simulink model "BalancingRobotSS"  (R2022b)
settings: Solver=ode15s  StartTime=0.0  StopTime=60  FixedStep=0.01  RelTol=1e-3
values from neighbouring files (symbols this model uses):
  drv =     [parameters.mat]
  gbox =     [parameters.mat]
  sens =     [parameters.mat]
  Ts = 1e-2    (= 0.01)    [DataLAB4.m]    (also in parameters.mat)
  wheel =     [parameters.mat]
undefined symbols (not defined in the file or in its folder): controller, DiscIntNeverNeededParam, filt, yaw
settings Model: Creator=Alessandro  LastModifiedBy=perondavid
settings SolverCC: AlgebraicLoopSolver=TrustRegion
settings ModelReferenceCC: EnableRefExpFcnMdlSchedulingChecks=on
settings RTWCC: DLArmComputeVersion=19.05

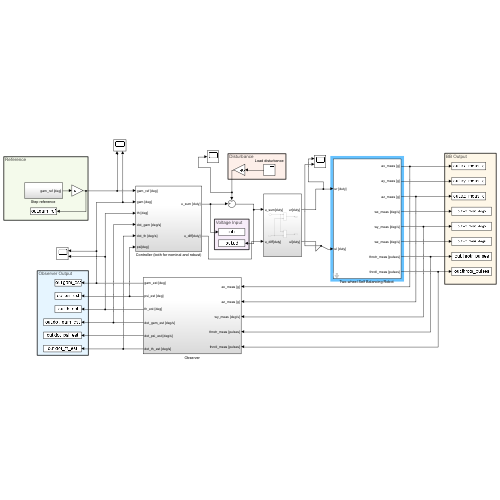
[thumbnail: Simulink's stored preview of the top-level diagram]
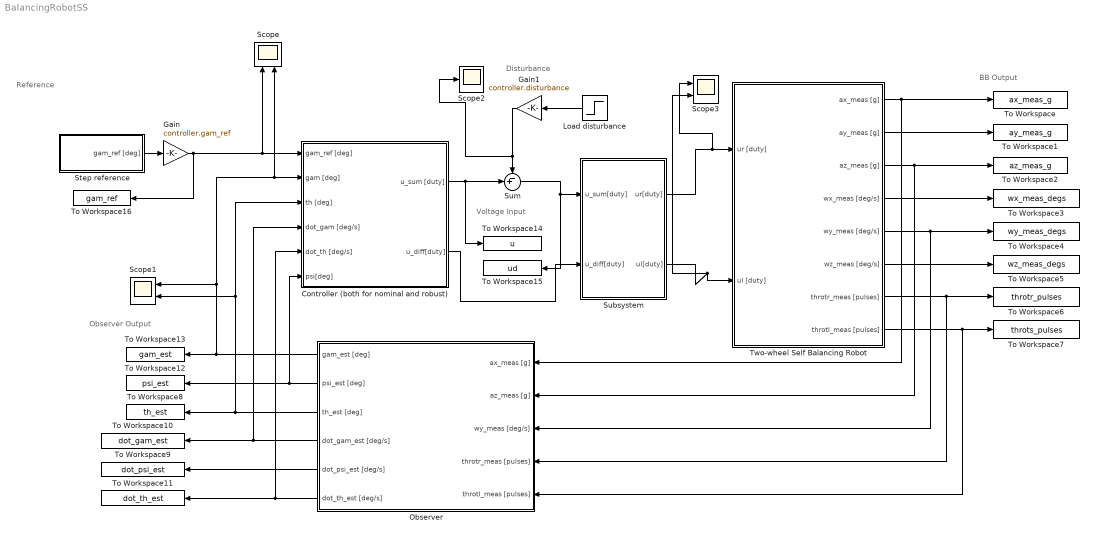
== system BalancingRobotSS ==
  note: Disturbance
  note: Reference
  note: Voltage Input
  note: Observer Output
  note: BB Output
  Controller (both for nominal and robust) : Subsystem
  Gain : Gain  Gain=controller.gam_ref
  Gain1 : Gain  Gain=controller.disturbance
  Load disturbance : Step  Time=10  After=5.0/drv.duty2V  SampleTime=Ts  VectorParams1D=off
  Observer : Subsystem
  Scope : Scope  NumInputPorts=2
  Scope1 : Scope  NumInputPorts=2
  Scope2 : Scope
  Scope3 : Scope  NumInputPorts=2
  "Step reference " : Subsystem
  Subsystem : Subsystem
  Sum : Sum  Inputs=-+|
  To Workspace : ToWorkspace  VariableName=ax_meas_g  SaveFormat=Structure With Time  SampleTime=-1
  To Workspace1 : ToWorkspace  VariableName=ay_meas_g  SaveFormat=Structure With Time  SampleTime=-1
  To Workspace10 : ToWorkspace  VariableName=dot_gam_est  SaveFormat=Structure With Time  SampleTime=-1
  To Workspace11 : ToWorkspace  VariableName=dot_th_est  SaveFormat=Structure With Time  SampleTime=-1
  To Workspace12 : ToWorkspace  VariableName=psi_est  SaveFormat=Structure With Time  SampleTime=-1
  To Workspace13 : ToWorkspace  VariableName=gam_est  SaveFormat=Structure With Time  SampleTime=-1
  To Workspace14 : ToWorkspace  VariableName=u  SaveFormat=Structure With Time  SampleTime=-1
  To Workspace15 : ToWorkspace  VariableName=ud  SaveFormat=Structure With Time  SampleTime=-1
  To Workspace16 : ToWorkspace  VariableName=gam_ref  SaveFormat=Structure With Time  SampleTime=-1
  To Workspace2 : ToWorkspace  VariableName=az_meas_g  SaveFormat=Structure With Time  SampleTime=-1
  To Workspace3 : ToWorkspace  VariableName=wx_meas_degs  SaveFormat=Structure With Time  SampleTime=-1
  To Workspace4 : ToWorkspace  VariableName=wy_meas_degs  SaveFormat=Structure With Time  SampleTime=-1
  To Workspace5 : ToWorkspace  VariableName=wz_meas_degs  SaveFormat=Structure With Time  SampleTime=-1
  To Workspace6 : ToWorkspace  VariableName=throtr_pulses  SaveFormat=Structure With Time  SampleTime=-1
  To Workspace7 : ToWorkspace  VariableName=throts_pulses  SaveFormat=Structure With Time  SampleTime=-1
  To Workspace8 : ToWorkspace  VariableName=th_est  SaveFormat=Structure With Time  SampleTime=-1
  To Workspace9 : ToWorkspace  VariableName=dot_psi_est  SaveFormat=Structure With Time  SampleTime=-1
  "Two-wheel Self Balancing Robot " : Subsystem  mask(Balancing robot (longitudinal + lateral dynamics)){initState=[0, 0, 0, 0, 0, 0], Ts=Ts}
      mask prompts: initState "Initial state [gam(0), psi(0), th(0), dot_gam(0), dot_psi(0), dot_th(0)]'"; Ts "Sample time:"
      mask help:
      | Balancing robot dynamic model.
      | Includes both the longitudinal and lateral (yaw) dynamics.
      mask init:
      | %% General parameters and conversion gains
      | 
      | %   gravity acc [m/s^2]
      | g = 9.81;
      | 
      | %   conversion gains
      | rpm2rads = 2*pi/60;         %   [rpm]   -> [rad/s]
      | rads2rpm = 60/2/pi;         %   [rad/s] -> [rpm]
      | rpm2degs = 360/60;          %   [rpm]   -> [deg/s]
      | degs2rpm = 60/360;          %   [deg/s] -> [rpm]
      | deg2rad = pi/180;           %   [deg]   -> [rad]
      | rad2deg = 180/pi;           %   [rad]   -> [deg]
      | g2ms2 = g;                  %   [acc_g] -> [m/s^2]
      | ms22g = 1/g;                %   [m/s^2] -> [acc_g]
      | ozin2Nm = 0.706e-2;         %   [oz*inch] -> [N*m]
      | 
      | 
      | %%  Battery data
      | 
      | %   electrical data
      | batt.UN = 11.1;     %   nominal voltage
      | 
      | 
      | %%  H-bridge PWM voltage driver
      | 
      | drv.Vbus = batt.UN;                     %   H-bridge DC bus voltage  
      | drv.pwm.bits = 8;                       %   PWM resolution [bits]
      | drv.pwm.levels = 2^drv.pwm.bits;        %   PWM levels
      | drv.pwm.Fs = 490;                       %   PWM frequency
      | drv.dutymax = drv.pwm.levels-1;         %   max duty cycle code
      | drv.duty2V = drv.Vbus/drv.dutymax;      %   duty cycle code (0-255) to voltage
      | drv.V2duty = drv.dutymax/drv.Vbus;      %   voltage to duty cycle code (0-255)
      | 
      | 
      | %%  Gearbox data 
      | 
      | gbox.N = 30;            %   reduction ratio
      | 
      | 
      | %%  Sensors data - Hall-effect encoder
      | 
      | %   Hall-effect encoder
      | sens.enc.ppr = 16*4;    %   pulses per rotation at motor side (w/ quadrature decoding)
      | sens.enc.pulse2deg = 360/sens.enc.ppr;
      | sens.enc.pulse2rad = 2*pi/sens.enc.ppr;
      | sens.enc.deg2pulse = sens.enc.ppr/360;
      | sens.enc.rad2pulse = sens.enc.ppr/2/pi;
      | 
      | 
      | %%  Sensors data - MPU6050 (accelerometer + gyro)
      | 
      | %   center of mass (CoM) position
      | sens.mpu.xb = 0;
      | sens.mpu.yb = 0;
      | sens.mpu.zb = 13.5e-3;
      | 
      | %       MPU6050 embedded accelerometer specs
      | sens.mpu.acc.bits = 16;
      | sens.mpu.acc.fs_g = 16;                                                         %   full-scale in "g" units
      | sens.mpu.acc.fs = sens.mpu.acc.fs_g * g2ms2;                                    %   full-scale in [m/s^2] 
      | sens.mpu.acc.g2LSB = floor(2^(sens.mpu.acc.bits-1)/sens.mpu.acc.fs_g);          %   sensitivity [LSB/g]
      | sens.mpu.acc.ms22LSB = sens.mpu.acc.g2LSB * ms22g;                              %   sensitvity [LSB/(m/s^2)]
      | sens.mpu.acc.LSB2g = sens.mpu.acc.fs_g/2^(sens.mpu.acc.bits-1);                 %   output quantization step [g/LSB]
      | sens.mpu.acc.LSB2ms2 = sens.mpu.acc.LSB2g * g2ms2;                              %   output quantization step [ms2/LSB]
      | sens.mpu.acc.bw = 94;                                                           %   output low-pass filter bandwidth
      | sens.mpu.acc.noisestd = 400e-6*sqrt(100);                                       %   output noise std [g-rms]
      | sens.mpu.acc.noisevar = sens.mpu.acc.noisestd^2;                                %   output noise var [g^2]
      | 
      | %       MPU6050 embdedded gyroscope specs
      | sens.mpu.gyro.bits = 16;
      | sens.mpu.gyro.fs_degs = 250;                                                    %   full scale in [deg/s (dps)]
      | sens.mpu.gyro.fs = sens.mpu.gyro.fs_degs * deg2rad;                             %   full scale in [rad/s]
      | sens.mpu.gyro.degs2LSB = floor(2^(sens.mpu.gyro.bits-1)/sens.mpu.gyro.fs_degs);	%   sensitivity [LSB/degs]
      | sens.mpu.gyro.rads2LSB = sens.mpu.gyro.degs2LSB * rad2deg;                      %   sensitivity [LSB/rads] 
      | sens.mpu.gyro.LSB2degs = sens.mpu.gyro.fs_degs/2^(sens.mpu.gyro.bits-1);        %   output quantization step [degs/LSB]
      | sens.mpu.gyro.LSB2rads = sens.mpu.gyro.LSB2degs * deg2rad;                      %   output quantization step [rads/LSB]
      | sens.mpu.gyro.bw = 98;                                                          %   output low-pass filter bandwidth
      | sens.mpu.gyro.noisestd = 5e-3*sqrt(100);                                        %   output noise std [degs-rms]
      | sens.mpu.gyro.noisevar = sens.mpu.acc.noisestd ^2;                              %   output noise var [degs^2]
      mask Help:
      | Riccardo Antonello (antonello@dei.unipd.it)
      | 
      | May 19, 2020
      | 
      | Dept. of Information Engineering, University of Padova
  wires:
  Controller (both for nominal and robust)/1(u_sum [duty]) -> To Workspace14/1, Sum/2
  Observer/1(gam_est [deg]) -> Scope1/1, Scope/2, Controller (both for nominal and robust)/2(gam [deg]), To Workspace13/1
  Sum/1 -> To Workspace15/1, Subsystem/1(u_sum[duty])
  "Two-wheel Self Balancing Robot "/2(ay_meas [g]) -> To Workspace1/1
  "Two-wheel Self Balancing Robot "/4(wx_meas [deg/s]) -> To Workspace3/1
  "Two-wheel Self Balancing Robot "/6(wz_meas [deg/s]) -> To Workspace5/1
  Observer/3(th_est [deg]) -> To Workspace8/1, Scope1/2, Controller (both for nominal and robust)/3(th [deg])
  Observer/6(dot_th_est [deg/s]) -> Controller (both for nominal and robust)/5(dot_th [deg/s]), To Workspace11/1
  Observer/5(dot_psi_est [deg/s]) -> To Workspace9/1
  Load disturbance/1 -> Gain1/1
  "Two-wheel Self Balancing Robot "/7(throtr_meas [pulses]) -> To Workspace6/1, Observer/4(throtr_meas [pulses])
  "Two-wheel Self Balancing Robot "/8(throtl_meas [pulses]) -> To Workspace7/1, Observer/5(throtl_meas [pulses])
  "Two-wheel Self Balancing Robot "/3(az_meas [g]) -> Observer/2(az_meas [g]), To Workspace2/1
  "Two-wheel Self Balancing Robot "/1(ax_meas [g]) -> Observer/1(ax_meas [g]), To Workspace/1
  "Two-wheel Self Balancing Robot "/5(wy_meas [deg/s]) -> To Workspace4/1, Observer/3(wy_meas [deg/s])
  Observer/4(dot_gam_est [deg/s]) -> Controller (both for nominal and robust)/4(dot_gam [deg/s]), To Workspace10/1
  Observer/2(psi_est [deg]) -> Controller (both for nominal and robust)/6(psi[deg]), To Workspace12/1
  Gain/1 -> To Workspace16/1, Scope/1, Controller (both for nominal and robust)/1(gam_ref [deg])
  Gain1/1 -> Sum/1, Scope2/1
  Controller (both for nominal and robust)/2(u_diff[duty]) -> Subsystem/2(u_diff[duty])
  Subsystem/1(ur[duty]) -> Scope3/1, "Two-wheel Self Balancing Robot "/1(ur [duty])
  Subsystem/2(ul[duty]) -> Scope3/2, "Two-wheel Self Balancing Robot "/2(ul [duty])
  "Step reference "/1(gam_ref [deg]) -> Gain/1

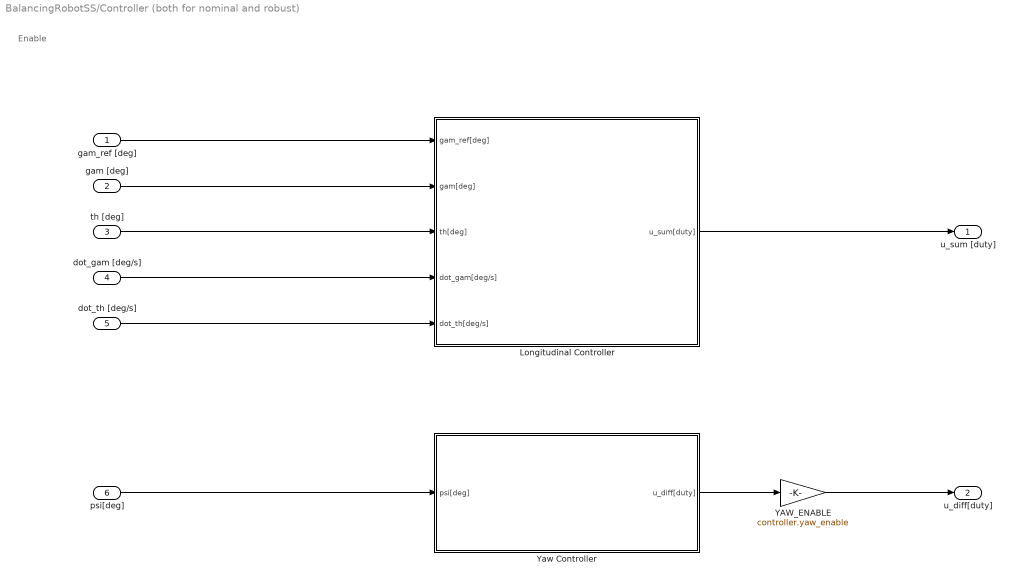
== system BalancingRobotSS/Controller (both for nominal and robust) ==
  note: Enable
  gam_ref [deg] : Inport
  gam [deg] : Inport  Port=2
  th [deg] : Inport  Port=3
  dot_gam [deg/s] : Inport  Port=4
  dot_th [deg/s] : Inport  Port=5
  psi[deg] : Inport  Port=6
  Longitudinal Controller : Subsystem
  YAW_ENABLE : Gain  Gain=controller.yaw_enable
  Yaw Controller : Subsystem
  u_sum [duty] : Outport
  u_diff[duty] : Outport  Port=2
  wires:
  psi[deg]/1 -> Yaw Controller/1(psi[deg])
  Yaw Controller/1(u_diff[duty]) -> YAW_ENABLE/1
  gam_ref [deg]/1 -> Longitudinal Controller/1(gam_ref[deg])
  gam [deg]/1 -> Longitudinal Controller/2(gam[deg])
  th [deg]/1 -> Longitudinal Controller/3(th[deg])
  dot_gam [deg/s]/1 -> Longitudinal Controller/4(dot_gam[deg/s])
  dot_th [deg/s]/1 -> Longitudinal Controller/5(dot_th[deg/s])
  Longitudinal Controller/1(u_sum[duty]) -> u_sum [duty]/1
  YAW_ENABLE/1 -> u_diff[duty]/1

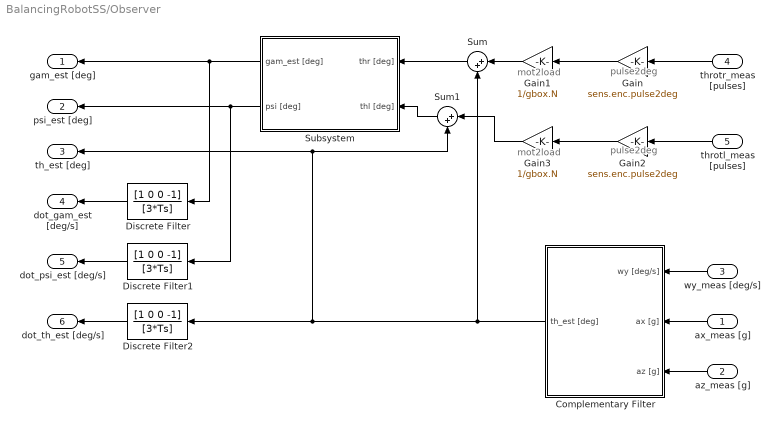
== system BalancingRobotSS/Observer ==
  note: mot2load
  note: pulse2deg
  note: mot2load
  note: pulse2deg
  ax_meas [g] : Inport
  az_meas [g] : Inport  Port=2
  wy_meas [deg/s] : Inport  Port=3
  throtr_meas [pulses] : Inport  Port=4
  throtl_meas [pulses] : Inport  Port=5
  Complementary Filter : Subsystem
  Discrete Filter : DiscreteFilter  Numerator=[1 0 0 -1]  Denominator=[3*Ts]  SampleTime=Ts
  Discrete Filter1 : DiscreteFilter  Numerator=[1 0 0 -1]  Denominator=[3*Ts]  SampleTime=Ts
  Discrete Filter2 : DiscreteFilter  Numerator=[1 0 0 -1]  Denominator=[3*Ts]  SampleTime=Ts
  Gain : Gain  Gain=sens.enc.pulse2deg
  Gain1 : Gain  Gain=1/gbox.N
  Gain2 : Gain  Gain=sens.enc.pulse2deg
  Gain3 : Gain  Gain=1/gbox.N
  Subsystem : Subsystem
  Sum : Sum  Inputs=|++
  Sum1 : Sum  Inputs=|++
  gam_est [deg] : Outport
  psi_est [deg] : Outport  Port=2
  th_est [deg] : Outport  Port=3
  dot_gam_est [deg/s] : Outport  Port=4
  dot_psi_est [deg/s] : Outport  Port=5
  dot_th_est [deg/s] : Outport  Port=6
  wires:
  Discrete Filter/1 -> dot_gam_est [deg/s]/1
  Gain1/1 -> Sum/1
  Discrete Filter1/1 -> dot_psi_est [deg/s]/1
  Gain/1 -> Gain1/1
  throtr_meas [pulses]/1 -> Gain/1
  wy_meas [deg/s]/1 -> Complementary Filter/1(wy [deg/s])
  Gain2/1 -> Gain3/1
  throtl_meas [pulses]/1 -> Gain2/1
  Gain3/1 -> Sum1/1
  Sum/1 -> Subsystem/1(thr [deg])
  Sum1/1 -> Subsystem/2(thl [deg])
  Complementary Filter/1(th_est [deg]) -> Sum1/2, th_est [deg]/1, Discrete Filter2/1, Sum/2
  Subsystem/2(psi [deg]) -> Discrete Filter1/1, psi_est [deg]/1
  Subsystem/1(gam_est [deg]) -> Discrete Filter/1, gam_est [deg]/1
  Discrete Filter2/1 -> dot_th_est [deg/s]/1
  ax_meas [g]/1 -> Complementary Filter/2(ax [g])
  az_meas [g]/1 -> Complementary Filter/3(az [g])

== system BalancingRobotSS/Step reference  ==
  Constant : Constant  Value=(0.1/wheel.r)*rad2deg
  gam_ref [deg] : Outport
  wires:
  Constant/1 -> gam_ref [deg]/1

== system BalancingRobotSS/Subsystem ==
  u_sum[duty] : Inport
  u_diff[duty] : Inport  Port=2
  Add : Sum
  Add1 : Sum  Inputs=+-
  ur[duty] : Outport
  ul[duty] : Outport  Port=2
  wires:
  u_diff[duty]/1 -> Add/2, Add1/2
  Add/1 -> ur[duty]/1
  u_sum[duty]/1 -> Add1/1, Add/1
  Add1/1 -> ul[duty]/1

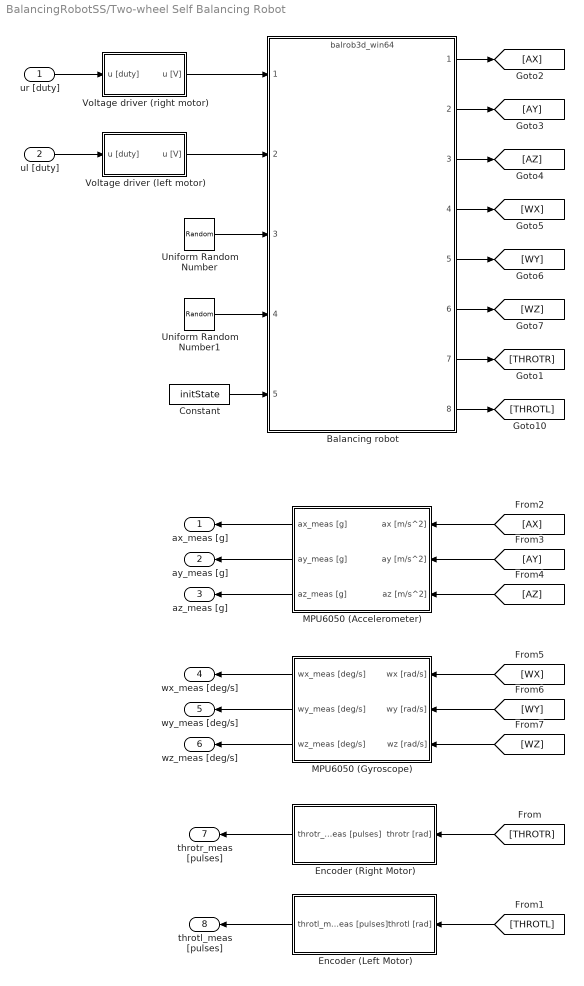
== system BalancingRobotSS/Two-wheel Self Balancing Robot  ==
  ur [duty] : Inport
  ul [duty] : Inport  Port=2
  Balancing robot : ModelReference  ModelNameDialog=balrob3d_win64.slxp  ModelReferenceVersion=1.741  CopyOfModelProtected=on
  Constant : Constant  Value=initState
  Encoder (Left Motor) : Subsystem
  Encoder (Right Motor) : Subsystem
  MPU6050 (Accelerometer) : Subsystem
  MPU6050 (Gyroscope) : Subsystem
  Uniform Random Number : UniformRandomNumber  Minimum=0.7  Maximum=1.3  SampleTime=1
  Uniform Random Number1 : UniformRandomNumber  Minimum=0.7  Maximum=1.3  Seed=10  SampleTime=1
  Voltage driver (left motor) : Subsystem
  Voltage driver (right motor) : Subsystem
  ax_meas [g] : Outport
  ay_meas [g] : Outport  Port=2
  az_meas [g] : Outport  Port=3
  wx_meas [deg/s] : Outport  Port=4
  wy_meas [deg/s] : Outport  Port=5
  wz_meas [deg/s] : Outport  Port=6
  throtr_meas [pulses] : Outport  Port=7
  throtl_meas [pulses] : Outport  Port=8
  wires:
  ur [duty]/1 -> Voltage driver (right motor)/1(u [duty])
  [WX] -> MPU6050 (Gyroscope)/1(wx [rad/s])
  Balancing robot/2 -> [AY]
  Balancing robot/4 -> [WX]
  Balancing robot/8 -> [THROTL]
  Balancing robot/1 -> [AX]
  [THROTL] -> Encoder (Left Motor)/1(throtl [rad])
  Balancing robot/6 -> [WZ]
  Balancing robot/7 -> [THROTR]
  Balancing robot/5 -> [WY]
  [AX] -> MPU6050 (Accelerometer)/1(ax [m/s^2])
  [WY] -> MPU6050 (Gyroscope)/2(wy [rad/s])
  Balancing robot/3 -> [AZ]
  [WZ] -> MPU6050 (Gyroscope)/3(wz [rad/s])
  [AZ] -> MPU6050 (Accelerometer)/3(az [m/s^2])
  [THROTR] -> Encoder (Right Motor)/1(throtr [rad])
  ul [duty]/1 -> Voltage driver (left motor)/1(u [duty])
  [AY] -> MPU6050 (Accelerometer)/2(ay [m/s^2])
  MPU6050 (Accelerometer)/1(ax_meas [g]) -> ax_meas [g]/1
  MPU6050 (Accelerometer)/2(ay_meas [g]) -> ay_meas [g]/1
  MPU6050 (Accelerometer)/3(az_meas [g]) -> az_meas [g]/1
  MPU6050 (Gyroscope)/1(wx_meas [deg/s]) -> wx_meas [deg/s]/1
  MPU6050 (Gyroscope)/2(wy_meas [deg/s]) -> wy_meas [deg/s]/1
  MPU6050 (Gyroscope)/3(wz_meas [deg/s]) -> wz_meas [deg/s]/1
  Encoder (Right Motor)/1(throtr_meas [pulses]) -> throtr_meas [pulses]/1
  Encoder (Left Motor)/1(throtl_meas [pulses]) -> throtl_meas [pulses]/1
  Voltage driver (right motor)/1(u [V]) -> Balancing robot/1
  Voltage driver (left motor)/1(u [V]) -> Balancing robot/2
  Uniform Random Number/1 -> Balancing robot/3
  Uniform Random Number1/1 -> Balancing robot/4
  Constant/1 -> Balancing robot/5

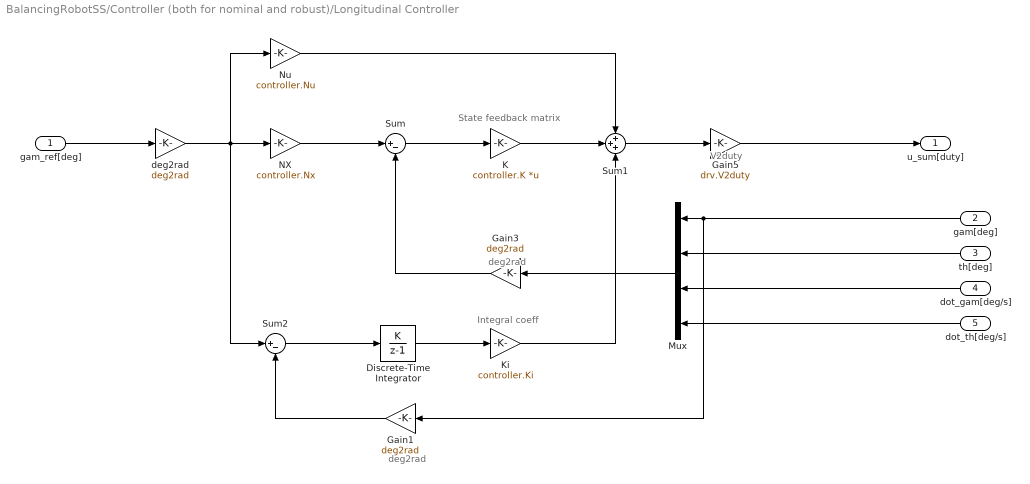
== system BalancingRobotSS/Controller (both for nominal and robust)/Longitudinal Controller ==
  note: State feedback matrix
  note: Integral coeff
  note: V2duty
  note: deg2rad
  note: deg2rad
  gam_ref[deg] : Inport
  gam[deg] : Inport  Port=2
  th[deg] : Inport  Port=3
  dot_gam[deg/s] : Inport  Port=4
  dot_th[deg/s] : Inport  Port=5
  Discrete-Time Integrator : DiscreteIntegrator  IntegratorMethod=Accumulation: Forward Euler  SampleTime=-1  ICPrevOutput=DiscIntNeverNeededParam  ICPrevScaledInput=DiscIntNeverNeededParam
  Gain1 : Gain  Gain=deg2rad
  Gain3 : Gain  Gain=deg2rad
  Gain5 : Gain  Gain=drv.V2duty
  K : Gain  Gain=controller.K  Multiplication=Matrix(K*u)
  Ki : Gain  Gain=controller.Ki
  Mux : Mux
  NX : Gain  Gain=controller.Nx
  Nu : Gain  Gain=controller.Nu
  Sum : Sum  Inputs=|+-
  Sum1 : Sum  Inputs=+++
  Sum2 : Sum  Inputs=|+-
  deg2rad : Gain  Gain=deg2rad
  u_sum[duty] : Outport
  wires:
  Discrete-Time Integrator/1 -> Ki/1
  dot_gam[deg/s]/1 -> Mux/3
  Sum2/1 -> Discrete-Time Integrator/1
  dot_th[deg/s]/1 -> Mux/4
  th[deg]/1 -> Mux/2
  gam_ref[deg]/1 -> deg2rad/1
  Ki/1 -> Sum1/3
  Nu/1 -> Sum1/1
  Gain5/1 -> u_sum[duty]/1
  Gain1/1 -> Sum2/2
  Mux/1 -> Gain3/1
  NX/1 -> Sum/1
  Sum1/1 -> Gain5/1
  Sum/1 -> K/1
  K/1 -> Sum1/2
  Gain3/1 -> Sum/2
  gam[deg]/1 -> Gain1/1, Mux/1
  deg2rad/1 -> NX/1, Nu/1, Sum2/1

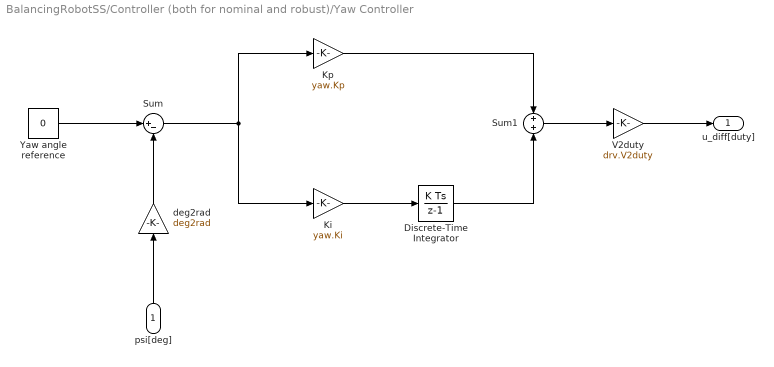
== system BalancingRobotSS/Controller (both for nominal and robust)/Yaw Controller ==
  psi[deg] : Inport
  Discrete-Time Integrator : DiscreteIntegrator  SampleTime=Ts  ICPrevOutput=DiscIntNeverNeededParam  ICPrevScaledInput=DiscIntNeverNeededParam
  Ki : Gain  Gain=yaw.Ki
  Kp : Gain  Gain=yaw.Kp
  Sum : Sum  Inputs=|+-
  Sum1 : Sum  Inputs=+|+
  V2duty : Gain  Gain=drv.V2duty
  Yaw angle reference : Constant  Value=0
  deg2rad : Gain  Gain=deg2rad
  u_diff[duty] : Outport
  wires:
  deg2rad/1 -> Sum/2
  psi[deg]/1 -> deg2rad/1
  Yaw angle reference/1 -> Sum/1
  Sum/1 -> Kp/1, Ki/1
  Sum1/1 -> V2duty/1
  V2duty/1 -> u_diff[duty]/1
  Kp/1 -> Sum1/1
  Discrete-Time Integrator/1 -> Sum1/2
  Ki/1 -> Discrete-Time Integrator/1

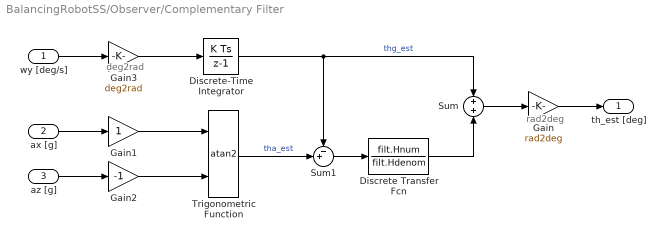
== system BalancingRobotSS/Observer/Complementary Filter ==
  note: rad2deg
  note: deg2rad
  wy [deg/s] : Inport
  ax [g] : Inport  Port=2
  az [g] : Inport  Port=3
  Discrete Transfer Fcn : DiscreteTransferFcn  Numerator=filt.Hnum  Denominator=filt.Hdenom  SampleTime=Ts
  Discrete-Time Integrator : DiscreteIntegrator  SampleTime=Ts  ICPrevOutput=DiscIntNeverNeededParam  ICPrevScaledInput=DiscIntNeverNeededParam
  Gain : Gain  Gain=rad2deg
  Gain1 : Gain
  Gain2 : Gain  Gain=-1
  Gain3 : Gain  Gain=deg2rad
  Sum : Sum  Inputs=+|+
  Sum1 : Sum  Inputs=-+|
  Trigonometric Function : Trigonometry  Operator=atan2
  th_est [deg] : Outport
  wires:
  Gain/1 -> th_est [deg]/1
  Sum/1 -> Gain/1
  ax [g]/1 -> Gain1/1
  Gain1/1 -> Trigonometric Function/1
  az [g]/1 -> Gain2/1
  Gain2/1 -> Trigonometric Function/2
  wy [deg/s]/1 -> Gain3/1
  Gain3/1 -> Discrete-Time Integrator/1
  Trigonometric Function/1 -> Sum1/2  "tha_est"
  Discrete-Time Integrator/1 -> Sum/1, Sum1/1  "thg_est"
  Sum1/1 -> Discrete Transfer Fcn/1
  Discrete Transfer Fcn/1 -> Sum/2

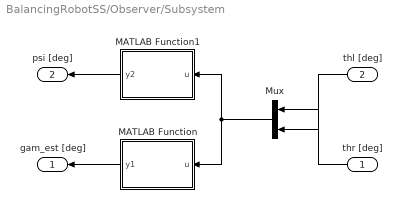
== system BalancingRobotSS/Observer/Subsystem ==
  thr [deg] : Inport
  thl [deg] : Inport  Port=2
  MATLAB Function : MATLAB Function  TreatAsAtomicUnit=on
  MATLAB Function1 : MATLAB Function  TreatAsAtomicUnit=on
  Mux : Mux  Inputs=2
  gam_est [deg] : Outport
  psi [deg] : Outport  Port=2
  wires:
  MATLAB Function1/1(y2) -> psi [deg]/1
  MATLAB Function/1(y1) -> gam_est [deg]/1
  Mux/1 -> MATLAB Function/1(u), MATLAB Function1/1(u)
  thr [deg]/1 -> Mux/1
  thl [deg]/1 -> Mux/2

== system BalancingRobotSS/Two-wheel Self Balancing Robot /Encoder (Left Motor) ==
  throtl [rad] : Inport
  Quantizer : Quantizer  QuantizationInterval=sens.enc.pulse2rad
  Zero-Order Hold : ZeroOrderHold  SampleTime=Ts
  rad2pulse : Gain  Gain=sens.enc.rad2pulse
  throtl_meas [pulses] : Outport
  wires:
  Quantizer/1 -> rad2pulse/1
  Zero-Order Hold/1 -> Quantizer/1
  throtl [rad]/1 -> Zero-Order Hold/1
  rad2pulse/1 -> throtl_meas [pulses]/1

== system BalancingRobotSS/Two-wheel Self Balancing Robot /Encoder (Right Motor) ==
  throtr [rad] : Inport
  Quantizer : Quantizer  QuantizationInterval=sens.enc.pulse2rad
  Zero-Order Hold : ZeroOrderHold  SampleTime=Ts
  rad2pulse : Gain  Gain=sens.enc.rad2pulse
  throtr_meas [pulses] : Outport
  wires:
  throtr [rad]/1 -> Zero-Order Hold/1
  Zero-Order Hold/1 -> Quantizer/1
  Quantizer/1 -> rad2pulse/1
  rad2pulse/1 -> throtr_meas [pulses]/1

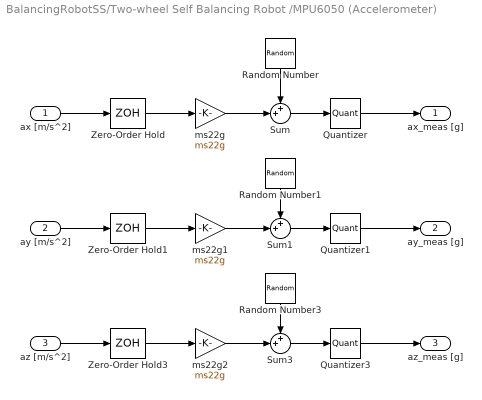
== system BalancingRobotSS/Two-wheel Self Balancing Robot /MPU6050 (Accelerometer) ==
  ax [m/s^2] : Inport
  ay [m/s^2] : Inport  Port=2
  az [m/s^2] : Inport  Port=3
  Quantizer : Quantizer  QuantizationInterval=sens.mpu.acc.LSB2g
  Quantizer1 : Quantizer  QuantizationInterval=sens.mpu.acc.LSB2g
  Quantizer3 : Quantizer  QuantizationInterval=sens.mpu.acc.LSB2g
  Random Number : RandomNumber  Variance=sens.mpu.acc.noisevar  Seed=1  SampleTime=Ts
  Random Number1 : RandomNumber  Variance=sens.mpu.acc.noisevar  Seed=10  SampleTime=Ts
  Random Number3 : RandomNumber  Variance=sens.mpu.acc.noisevar  Seed=100  SampleTime=Ts
  Sum : Sum  Inputs=++|
  Sum1 : Sum  Inputs=++|
  Sum3 : Sum  Inputs=++|
  Zero-Order Hold : ZeroOrderHold  SampleTime=Ts
  Zero-Order Hold1 : ZeroOrderHold  SampleTime=Ts
  Zero-Order Hold3 : ZeroOrderHold  SampleTime=Ts
  ms22g : Gain  Gain=ms22g
  ms22g1 : Gain  Gain=ms22g
  ms22g2 : Gain  Gain=ms22g
  ax_meas [g] : Outport
  ay_meas [g] : Outport  Port=2
  az_meas [g] : Outport  Port=3
  wires:
  ax [m/s^2]/1 -> Zero-Order Hold/1
  Zero-Order Hold1/1 -> ms22g1/1
  Sum1/1 -> Quantizer1/1
  ms22g/1 -> Sum/2
  ay [m/s^2]/1 -> Zero-Order Hold1/1
  Sum3/1 -> Quantizer3/1
  ms22g1/1 -> Sum1/2
  Random Number1/1 -> Sum1/1
  Random Number/1 -> Sum/1
  Sum/1 -> Quantizer/1
  Random Number3/1 -> Sum3/1
  ms22g2/1 -> Sum3/2
  Zero-Order Hold3/1 -> ms22g2/1
  az [m/s^2]/1 -> Zero-Order Hold3/1
  Zero-Order Hold/1 -> ms22g/1
  Quantizer/1 -> ax_meas [g]/1
  Quantizer1/1 -> ay_meas [g]/1
  Quantizer3/1 -> az_meas [g]/1

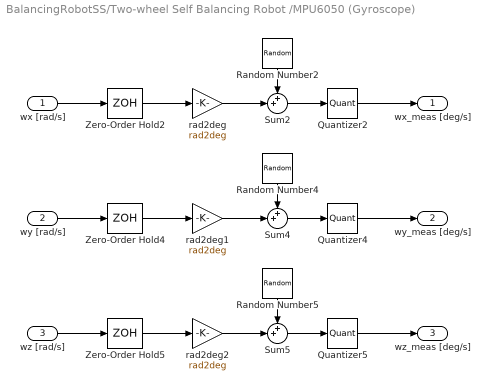
== system BalancingRobotSS/Two-wheel Self Balancing Robot /MPU6050 (Gyroscope) ==
  wx [rad/s] : Inport
  wy [rad/s] : Inport  Port=2
  wz [rad/s] : Inport  Port=3
  Quantizer2 : Quantizer  QuantizationInterval=sens.mpu.gyro.LSB2degs
  Quantizer4 : Quantizer  QuantizationInterval=sens.mpu.gyro.LSB2degs
  Quantizer5 : Quantizer  QuantizationInterval=sens.mpu.gyro.LSB2degs
  Random Number2 : RandomNumber  Variance=sens.mpu.gyro.noisevar  Seed=2  SampleTime=Ts
  Random Number4 : RandomNumber  Variance=sens.mpu.gyro.noisevar  Seed=20  SampleTime=Ts
  Random Number5 : RandomNumber  Variance=sens.mpu.gyro.noisevar  Seed=200  SampleTime=Ts
  Sum2 : Sum  Inputs=++|
  Sum4 : Sum  Inputs=++|
  Sum5 : Sum  Inputs=++|
  Zero-Order Hold2 : ZeroOrderHold  SampleTime=Ts
  Zero-Order Hold4 : ZeroOrderHold  SampleTime=Ts
  Zero-Order Hold5 : ZeroOrderHold  SampleTime=Ts
  rad2deg : Gain  Gain=rad2deg
  rad2deg1 : Gain  Gain=rad2deg
  rad2deg2 : Gain  Gain=rad2deg
  wx_meas [deg/s] : Outport
  wy_meas [deg/s] : Outport  Port=2
  wz_meas [deg/s] : Outport  Port=3
  wires:
  Random Number2/1 -> Sum2/1
  Sum2/1 -> Quantizer2/1
  Quantizer2/1 -> wx_meas [deg/s]/1
  Zero-Order Hold5/1 -> rad2deg2/1
  Sum4/1 -> Quantizer4/1
  rad2deg/1 -> Sum2/2
  rad2deg2/1 -> Sum5/2
  Random Number5/1 -> Sum5/1
  Zero-Order Hold4/1 -> rad2deg1/1
  Sum5/1 -> Quantizer5/1
  Random Number4/1 -> Sum4/1
  Zero-Order Hold2/1 -> rad2deg/1
  Quantizer5/1 -> wz_meas [deg/s]/1
  wz [rad/s]/1 -> Zero-Order Hold5/1
  wx [rad/s]/1 -> Zero-Order Hold2/1
  rad2deg1/1 -> Sum4/2
  Quantizer4/1 -> wy_meas [deg/s]/1
  wy [rad/s]/1 -> Zero-Order Hold4/1

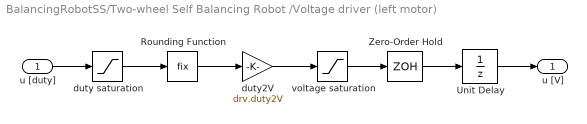
== system BalancingRobotSS/Two-wheel Self Balancing Robot /Voltage driver (left motor) ==
  u [duty] : Inport
  Rounding Function : Rounding  Operator=fix
  Unit Delay : UnitDelay  SampleTime=1/drv.pwm.Fs  HasFrameUpgradeWarning=on
  Zero-Order Hold : ZeroOrderHold  SampleTime=Ts
  duty saturation : Saturate  UpperLimit=255  LowerLimit=-255
  duty2V : Gain  Gain=drv.duty2V
  voltage saturation : Saturate  UpperLimit=drv.Vbus  LowerLimit=-drv.Vbus
  u [V] : Outport
  wires:
  Zero-Order Hold/1 -> Unit Delay/1
  u [duty]/1 -> duty saturation/1
  voltage saturation/1 -> Zero-Order Hold/1
  duty saturation/1 -> Rounding Function/1
  Rounding Function/1 -> duty2V/1
  duty2V/1 -> voltage saturation/1
  Unit Delay/1 -> u [V]/1

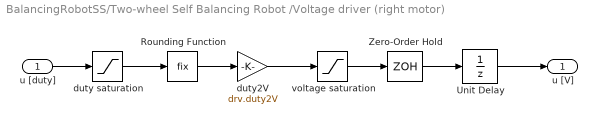
== system BalancingRobotSS/Two-wheel Self Balancing Robot /Voltage driver (right motor) ==
  u [duty] : Inport
  Rounding Function : Rounding  Operator=fix
  Unit Delay : UnitDelay  SampleTime=1/drv.pwm.Fs  HasFrameUpgradeWarning=on
  Zero-Order Hold : ZeroOrderHold  SampleTime=Ts
  duty saturation : Saturate  UpperLimit=255  LowerLimit=-255
  duty2V : Gain  Gain=drv.duty2V
  voltage saturation : Saturate  UpperLimit=drv.Vbus  LowerLimit=-drv.Vbus
  u [V] : Outport
  wires:
  u [duty]/1 -> duty saturation/1
  duty saturation/1 -> Rounding Function/1
  Zero-Order Hold/1 -> Unit Delay/1
  voltage saturation/1 -> Zero-Order Hold/1
  Rounding Function/1 -> duty2V/1
  duty2V/1 -> voltage saturation/1
  Unit Delay/1 -> u [V]/1

== matlab function BalancingRobotSS/Observer/Subsystem/MATLAB Function ==
  data: u input; y1 output
function y1 = gam_angle(u)

y1=(u(1)+u(2))/2;

== matlab function BalancingRobotSS/Observer/Subsystem/MATLAB Function1 ==
  data: u input; y2 output
function y2 = psi_angle(u)
wheel.r = 0.034;
wheel.yb=0.1;
w=2*abs(wheel.yb);

y2 = (wheel.r/w)*(u(1)-u(2));
